simulink model "MPC_testing"  (R2014b)
settings: Solver=ode45  StartTime=0.0  StopTime=30  RelTol=1e-3
StopFcn:
  | plotting
settings Model: Creator=danielpihlquist  LastModifiedBy=danielpihlquist
settings DebuggingCC: SignalLabelMismatchMsg=warning  SFcnCompatibilityMsg=warning  StrictBusMsg=WarnOnBusTreatedAsVector  NonBusSignalsTreatedAsBus=warning

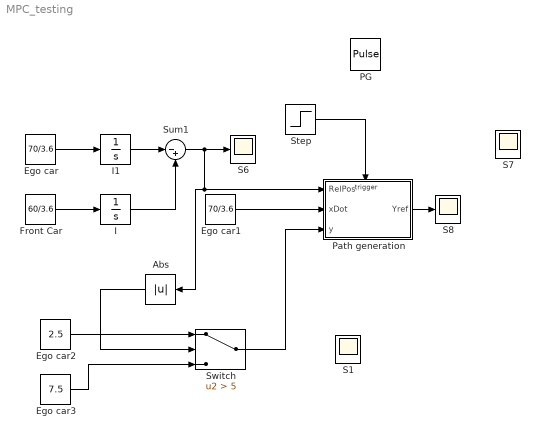
== system MPC_testing ==
  Abs : Abs
  Ego car : Constant  Value=70/3.6
  Ego car1 : Constant  Value=70/3.6
  Ego car2 : Constant  Value=2.5
  Ego car3 : Constant  Value=7.5
  Front Car : Constant  Value=60/3.6
  I : Integrator  InitialCondition=70
  I1 : Integrator
  PG : DiscretePulseGenerator  PulseType=Time based  Period=3  PulseWidth=5
  Path generation : Subsystem
  S{1,6..8} (4 alike) : Scope
      S1 settings: YMin=0  YMax=9
      S6 settings: YMin=0  YMax=9  SaveName=ScopeData8
      S7 settings: YMin=0  YMax=9  SaveName=ScopeData9
      S8 settings: YMin=0  YMax=9  SaveName=ScopeData10
  Step : Step  Time=0.00001  SampleTime=0
  Sum1 : Sum  Inputs=|-+
  Switch : Switch  Criteria=u2 > Threshold  Threshold=5
  wires:
  Front Car/1 -> I/1
  Path generation/1(Yref) -> S8/1
  I/1 -> Sum1/2
  Sum1/1 -> Path generation/1(RelPos), Abs/1, S6/1
  Ego car/1 -> I1/1
  I1/1 -> Sum1/1
  Ego car1/1 -> Path generation/2(xDot)
  Ego car2/1 -> Switch/1
  Ego car3/1 -> Switch/3
  Abs/1 -> Switch/2
  Switch/1 -> Path generation/3(y)
  Step/1 -> Path generation/Trigger

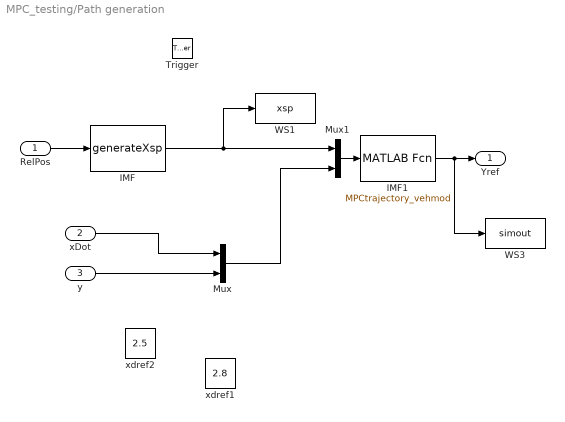
== system MPC_testing/Path generation ==
  RelPos : Inport
  xDot : Inport  Port=2
  y : Inport  Port=3
  Trigger : TriggerPort  PortDimensions=1
  IMF : MATLABFcn  MATLABFcn=generateXsp
  IMF1 : MATLABFcn  MATLABFcn=MPCtrajectory_vehmod
  Mux : Mux  Inputs=2
  Mux1 : Mux  Inputs=2
  WS1 : ToWorkspace  VariableName=xsp  SampleTime=-1
  WS3 : ToWorkspace  VariableName=simout  SampleTime=-1
  xdref1 : Constant  Value=2.8
  xdref2 : Constant  Value=2.5
  Yref : Outport
  wires:
  Mux1/1 -> IMF1/1
  IMF1/1 -> WS3/1, Yref/1
  Mux/1 -> Mux1/2
  IMF/1 -> WS1/1, Mux1/1
  RelPos/1 -> IMF/1
  y/1 -> Mux/2
  xDot/1 -> Mux/1
